simulink model "ansiBPF"  (R2018a)
settings: Solver=VariableStepAuto  StartTime=0.0  StopTime=0.001  RelTol=1e-3
undefined symbols (not defined in the file): fdesignblkfcn, G1, G10, G11, G12, G13, G14, G15, G16, G17, G18, G19, G2, G20, G21, G22, G23, G24, G25, G26, G3, G4, G5, G6, G7, G8, G9, gcbh, get, T
libraries: dspsrcs4 x1, dspxfrm3 x1, dspobslib x1
(part 4 of 8)

== system ansiBPF/Filter Bank /Filter 2/Bandpass Filter ==
  In : Inport
  Generated Filter Block : DiscreteFir  Tag=BlockMethodSubSystem  Coefficients=[-0.0065520904327652698 -0.00010517582880906067 -0.000106202106848731628 -0.000106471335176881615 -0.000107477567639228551 -0.000107717034781466795 -0.000108707029335038306 -0.000108916686469714039 -0.000109893182034219688 -0.000110062510787145129 -0.00011102648219109485 -0.000111156921073082989 -0.000112107487192741569 -0.000112182333314063312 -0.000113126641755007521 -0.000113131885304980148 -0.000114064527094245025 -0.000113984309255005527 -0.000114903486523693397 -0.000114709259579534573 -0.00011560471702884213 -0.000115250498002208749 -0.000116118499658339445 -0.000115523438953155764 -0.000116352882639977355 -0.000115401368602836474 -0.000116178949793126728 -0.000114624497724521529 -0.000115369912653134232 -0.000112588103045363787 -0.000113454382439510143 -0.000105600047188595213 -0.000119601086627533416 -0.000118265326543747656 -0.000113707630059844983 -0.000115245875398465453 -0.000113542007242014353 -0.000114206276410826964 -0.000113038053698082558 -0.000113288140558110781 -0.000112317213569619931 -0.000112298715604786041 -0.000111401966908671699 -0.00011118586931709082 -0.000110317490532845457 -0.000109931475373507568 -0.000109068923417750732 -0.00010854161052693912 -0.000107671085028851181 -0.00010702232303319021 -0.000106149481673625603 -0.000105400716505062923 -0.000104538776781785522 -0.000103701435228590379 -0.00010287976398070452 -0.000101959768047119913 -0.000101195692603928266 -0.000100186936410765355 -9.95035075239295388e-05 -9.83174158083373339e-05 -9.77096772610169036e-05 -9.60390900783103095e-05 -9.54411628696673884e-05 -9.12570311761172812e-05 -9.07561017200339494e-05 -9.18203001805116987e-05 -8.88167101968278855e-05 -8.82725884827313472e-05 -8.61803095726835599e-05 -8.52455091440471957e-05 -8.33066481701604666e-05 -8.21629941521981354e-05 -8.02634435504320608e-05 -7.89730436054292625e-05 -7.70623249042409373e-05 -7.56461343801691157e-05 -7.37098559646547823e-05 -7.21736889675037095e-05 -7.01902107722095176e-05 -6.85411372962618364e-05 -6.64933063759829757e-05 -6.47234785814985243e-05 -6.25988149661926065e-05 -6.07047494799575136e-05 -5.85014502508473085e-05 -5.64763675034889233e-05 -5.42061958653215431e-05 -5.2069028066990842e-05 -4.97523995651258122e-05 -4.75377184257138395e-05 -4.52500612704045846e-05 -4.30099879797583626e-05 -4.08564766485516726e-05 -3.86131768993000564e-05 -3.67249383764373815e-05 -3.37927058845015983e-05 -2.99702146047041205e-05 -2.88591967940549146e-05 -2.5643989191950348e-05 -2.33889216439079105e-05 -2.03913616446912292e-05 -1.79432200990902943e-05 -1.49369061498760619e-05 -1.23551713843077239e-05 -9.30436837727774398e-06 -6.6191240498310674e-06 -3.51263187217327546e-06 -7.29210176946567054e-07 2.42943627883229804e-06 5.29608805909416718e-06 8.51213489002973798e-06 1.14495124214844151e-05 1.47183609002235807e-05 1.77261107676888167e-05 2.10528312953355682e-05 2.41378812306237166e-05 2.75284516797371758e-05 3.07100728408501346e-05 3.41889814983957266e-05 3.74783404359386516e-05 4.10725051253248711e-05 4.44933876151153477e-05 4.819528456261501e-05 5.17150159014216813e-05 5.54485610139596617e-05 5.89203449214868716e-05 6.24089364694020948e-05 6.54624198478557319e-05 7.02950922839306095e-05 7.35151336678137866e-05 7.74448122048125467e-05 8.1119897301276176e-05 8.50901267330924179e-05 8.88362903187010062e-05 9.28611303475984553e-05 9.66774420023970679e-05 0.000100766015137432097 0.000104648455574905347 0.000108797922116939943 0.000112754457292972638 0.000116969485745546133 0.00012099177234329054 0.000125276120152343273 0.000129360951804791038 0.00013370205653710524 0.000137838696799424791 0.000142224618045109244 0.000146402778520629919 0.000150816605519575169 0.000155021842835372572 0.000159469307385238601 0.000163695674996933887 0.000168189260407265316 0.000172476265056720597 0.000177067943764805825 0.000181458287998302164 0.000186203754671019489 0.000190675143679076137 0.000195459625813089487 0.000199289859472990291 0.00020433802273071692 0.000208929741926855244 ...(+38651 chars)]  InputProcessing=Columns as channels (frame based)
  Out : Outport
  wires:
  In/1 -> Generated Filter Block/1
  Generated Filter Block/1 -> Out/1

== system ansiBPF/Filter Bank /Filter 20/Bandpass Filter ==
  In : Inport
  Generated Filter Block : DiscreteFir  Tag=BlockMethodSubSystem  Coefficients=[-0.00113497349630124365 -0.00144460007081206572 -0.00133761993915687809 -0.000286951069466899271 0.00144271591023053961 0.00300366183089492266 0.00342621926386496144 0.00232618430369092247 0.000355941340853791182 -0.00106524193379941147 -0.000764417441251011298 0.00104125888033931163 0.00238356782823430499 0.000563114599062660998 -0.00575231519277760554 -0.0146223238558608748 -0.02068934809150412 -0.017570022993308218 -0.0019647947130488853 0.0228074696890188111 0.0464246679115413105 0.0555114348337037294 0.0405989235530393386 0.00255852110341019644 -0.0454472973928045851 -0.0825056954461215186 -0.0895173822287154697 -0.0592064535996665031 -0.00117072147033643256 0.0612447115066645995 0.101265296297444102 0.101265296297444102 0.0612447115066645995 -0.00117072147033643256 -0.0592064535996665031 -0.0895173822287154697 -0.0825056954461215186 -0.0454472973928045851 0.00255852110341019644 0.0405989235530393386 0.0555114348337037294 0.0464246679115413105 0.0228074696890188111 -0.0019647947130488853 -0.017570022993308218 -0.02068934809150412 -0.0146223238558608748 -0.00575231519277760554 0.000563114599062660998 0.00238356782823430499 0.00104125888033931163 -0.000764417441251011298 -0.00106524193379941147 0.000355941340853791182 0.00232618430369092247 0.00342621926386496144 0.00300366183089492266 0.00144271591023053961 -0.000286951069466899271 -0.00133761993915687809 -0.00144460007081206572 -0.00113497349630124365]  InputProcessing=Columns as channels (frame based)
  Out : Outport
  wires:
  In/1 -> Generated Filter Block/1
  Generated Filter Block/1 -> Out/1

== system ansiBPF/Filter Bank /Filter 21/Bandpass Filter ==
  In : Inport
  Generated Filter Block : DiscreteFir  Tag=BlockMethodSubSystem  Coefficients=[0.00137967792408118586 0.00203511795884510956 0.00128120156665517378 -0.00101589038743776566 -0.00281172473857506681 -0.00206474565505353289 -4.06895703725833682e-06 -0.00124668179767388866 -0.00848684238187791436 -0.0161658520413711648 -0.0116221923225929107 0.0130472223023156003 0.0474189814395482231 0.0630804183485078329 0.0342498131107656437 -0.0351459615027731181 -0.103660410808636957 -0.117606073858950277 -0.0540457344117714067 0.0542059776584169067 0.136793566102791558 0.136793566102791558 0.0542059776584169067 -0.0540457344117714067 -0.117606073858950277 -0.103660410808636957 -0.0351459615027731181 0.0342498131107656437 0.0630804183485078329 0.0474189814395482231 0.0130472223023156003 -0.0116221923225929107 -0.0161658520413711648 -0.00848684238187791436 -0.00124668179767388866 -4.06895703725833682e-06 -0.00206474565505353289 -0.00281172473857506681 -0.00101589038743776566 0.00128120156665517378 0.00203511795884510956 0.00137967792408118586]  InputProcessing=Columns as channels (frame based)
  Out : Outport
  wires:
  In/1 -> Generated Filter Block/1
  Generated Filter Block/1 -> Out/1

== system ansiBPF/Filter Bank /Filter 22/Bandpass Filter ==
  In : Inport
  Generated Filter Block : DiscreteFir  Tag=BlockMethodSubSystem  Coefficients=[-0.000239399053005650463 0.00157980635298882654 0.00273914312615368503 0.000923834018831144656 -0.00211907071210376639 -0.00123704307828366184 0.00141073161762023374 -0.00525586180253685611 -0.0212063774776766259 -0.020538553956489191 0.020363405111988999 0.0736808944472505389 0.0675221257088605281 -0.0277428030971744559 -0.133457100793600208 -0.126756290889779882 0.0133480541137937919 0.157477448437687739 0.157477448437687739 0.0133480541137937919 -0.126756290889779882 -0.133457100793600208 -0.0277428030971744559 0.0675221257088605281 0.0736808944472505389 0.020363405111988999 -0.020538553956489191 -0.0212063774776766259 -0.00525586180253685611 0.00141073161762023374 -0.00123704307828366184 -0.00211907071210376639 0.000923834018831144656 0.00273914312615368503 0.00157980635298882654 -0.000239399053005650463]  InputProcessing=Columns as channels (frame based)
  Out : Outport
  wires:
  In/1 -> Generated Filter Block/1
  Generated Filter Block/1 -> Out/1

== system ansiBPF/Filter Bank /Filter 23/Bandpass Filter ==
  In : Inport
  Generated Filter Block : DiscreteFir  Tag=BlockMethodSubSystem  Coefficients=[0.0016036920117646358 -0.000136506919232390371 -0.00554654416115776643 -0.00409854373436943295 0.00651234636097152916 0.0086281924311640678 -0.000812948820277657942 0.000616255127543447281 0.00485788280046386359 -0.0231134611060915159 -0.0454776771227874202 0.0199173964444624811 0.110386701196003828 0.0492000037752856126 -0.132302802697052024 -0.155676573956482767 0.0607793504320709513 0.208466790714563727 0.0607793504320709513 -0.155676573956482767 -0.132302802697052024 0.0492000037752856126 0.110386701196003828 0.0199173964444624811 -0.0454776771227874202 -0.0231134611060915159 0.00485788280046386359 0.000616255127543447281 -0.000812948820277657942 0.0086281924311640678 0.00651234636097152916 -0.00409854373436943295 -0.00554654416115776643 -0.000136506919232390371 0.0016036920117646358]  InputProcessing=Columns as channels (frame based)
  Out : Outport
  wires:
  In/1 -> Generated Filter Block/1
  Generated Filter Block/1 -> Out/1

== system ansiBPF/Filter Bank /Filter 24/Bandpass Filter ==
  In : Inport
  Generated Filter Block : DiscreteFir  Tag=BlockMethodSubSystem  Coefficients=[0.00173845719790115044 -0.00208182224518605862 -0.00633078104393082659 0.00570355342010059677 0.0118157687154328388 -0.00910426009286301359 -0.0127800340964993719 0.00633831045103573198 0.00108790409523717036 0.00960173909386747258 0.0284652419898162971 -0.0422562821460850044 -0.0728901496183085584 0.0868874680296221752 0.119563090778747619 -0.130057123194459334 -0.151259951570923645 0.155157286338985317 0.155157286338985317 -0.151259951570923645 -0.130057123194459334 0.119563090778747619 0.0868874680296221752 -0.0728901496183085584 -0.0422562821460850044 0.0284652419898162971 0.00960173909386747258 0.00108790409523717036 0.00633831045103573198 -0.0127800340964993719 -0.00910426009286301359 0.0118157687154328388 0.00570355342010059677 -0.00633078104393082659 -0.00208182224518605862 0.00173845719790115044]  InputProcessing=Columns as channels (frame based)
  Out : Outport
  wires:
  In/1 -> Generated Filter Block/1
  Generated Filter Block/1 -> Out/1
